simulink model "plant_model"  (R2023b)
settings: Solver=VariableStepAuto  StartTime=0.0  StopTime=10.0  RelTol=1e-3
values from neighbouring files (symbols this model uses):
  K = 6.2    [CA3_params.m]    (also in CA3_params_integral.m; CA3_params_yp.m)
  K_theta = 36    [CA3_params.m]    (also in CA3_params_integral.m; CA3_params_yp.m)
  K_w = 0.7827563    [CA3_params.m]    (also in CA3_params_integral.m; CA3_params_yp.m)
  tau = 0.25    [CA3_params.m]    (also in CA3_params_integral.m; CA3_params_yp.m)
settings Model: Creator=john  LastModifiedBy=john

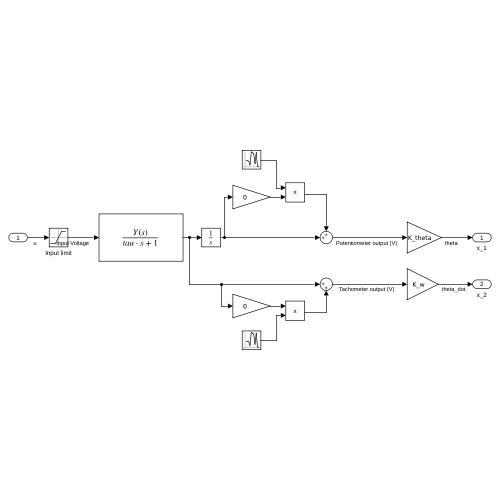
[thumbnail: Simulink's stored preview of the top-level diagram]
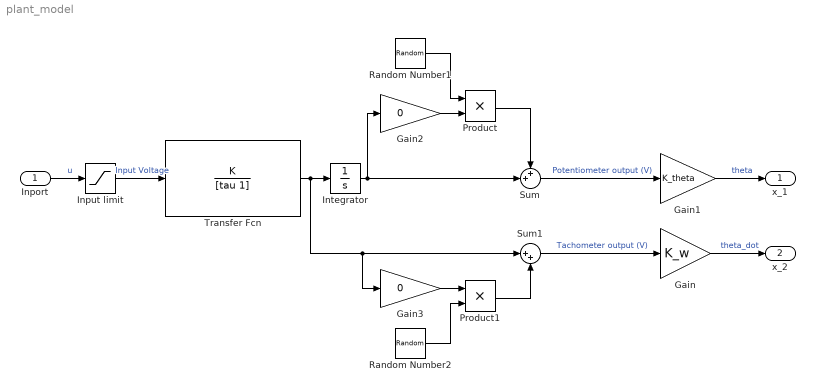
== system plant_model ==
  Inport : Inport
  Gain : Gain  Gain=K_w
  Gain1 : Gain  Gain=K_theta
  Gain2 : Gain  Gain=0
  Gain3 : Gain  Gain=0
  Input limit : Saturate  UpperLimit=5  LowerLimit=-5
  Integrator : Integrator
  Product : Product
  Product1 : Product
  Random Number1 : RandomNumber  SampleTime=0.1
  Random Number2 : RandomNumber  SampleTime=0.1
  Sum : Sum  Inputs=++|
  Sum1 : Sum  Inputs=|++
  Transfer Fcn : TransferFcn  Numerator=K  Denominator=[tau 1]
  x_1 : Outport
  x_2 : Outport  Port=2
  wires:
  Inport/1 -> Input limit/1  "u"
  Integrator/1 -> Sum/2, Gain2/1
  Gain/1 -> x_2/1  "theta_dot"
  Gain1/1 -> x_1/1  "theta"
  Input limit/1 -> Transfer Fcn/1  "Input Voltage"
  Sum1/1 -> Gain/1  "Tachometer output (V)"
  Random Number1/1 -> Product/1
  Sum/1 -> Gain1/1  "Potentiometer output (V)"
  Gain2/1 -> Product/2
  Product/1 -> Sum/1
  Random Number2/1 -> Product1/2
  Product1/1 -> Sum1/2
  Transfer Fcn/1 -> Integrator/1, Sum1/1, Gain3/1
  Gain3/1 -> Product1/1
